simulink model "scheme2"  (R2024a)
settings: Solver=VariableStepAuto  StartTime=0.0  StopTime=10.0  RelTol=1e-8
values from neighbouring files (symbols this model uses):
  A = [8, 1, 11; 4, 0, 4; -4, -3, -7]    [main.m]
  B = [-1; -3; 3]    [main.m]
  Cz = [-2, -3, -1]    [main.m]
  Dz = [8, -8, 12, -3]    [main.m]
  Gamma = [-40, 16, 9, 7; -64, 25, 14, 12; -26, 11, 7, 3; -48, 18, 14, 8]    [main.m]
  K1 = [0, 0, 0]    [main.m]
  K2 = FindFeedforwardController(A, B, Gamma, Cz, Dz, zeros(3, 4), K1)    [main.m]
  wgen = 1    [main.m]
  x0 = [1; 1; 1]    [main.m]
settings Model: Creator=alexivanov  LastModifiedBy=alexivanov

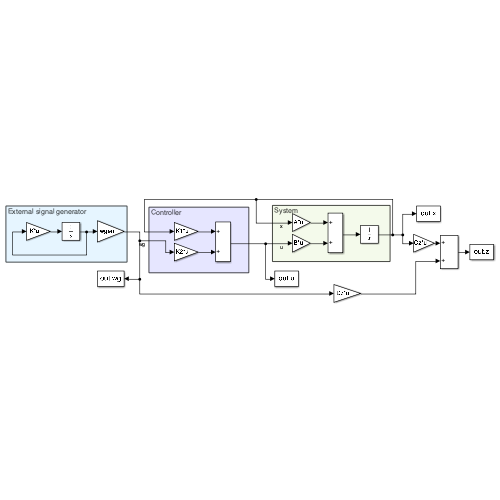
[thumbnail: Simulink's stored preview of the top-level diagram]
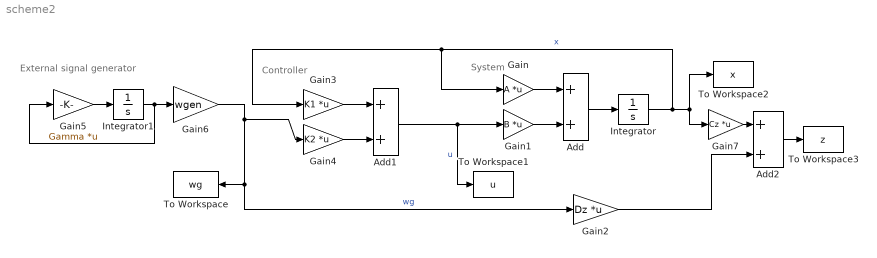
== system scheme2 ==
  note: Controller
  note: External signal generator
  note: System
  Add : Sum
  Add1 : Sum
  Add2 : Sum
  Gain : Gain  Gain=A  Multiplication=Matrix(K*u)
  Gain1 : Gain  Gain=B  Multiplication=Matrix(K*u)
  Gain2 : Gain  Gain=Dz  Multiplication=Matrix(K*u)
  Gain3 : Gain  Gain=K1  Multiplication=Matrix(K*u)
  Gain4 : Gain  Gain=K2  Multiplication=Matrix(K*u)
  Gain5 : Gain  Gain=Gamma  Multiplication=Matrix(K*u)
  Gain6 : Gain  Gain=wgen
  Gain7 : Gain  Gain=Cz  Multiplication=Matrix(K*u)
  Integrator : Integrator  InitialCondition=x0
  Integrator1 : Integrator  InitialCondition=[1; 1; 1; 1]
  To Workspace : ToWorkspace  VariableName=wg  SampleTime=-1
  To Workspace1 : ToWorkspace  VariableName=u  SampleTime=-1
  To Workspace2 : ToWorkspace  VariableName=x  SampleTime=-1
  To Workspace3 : ToWorkspace  VariableName=z  SampleTime=-1
  wires:
  Add/1 -> Integrator/1
  Gain/1 -> Add/1
  Integrator/1 -> Gain7/1, To Workspace2/1, Gain3/1, Gain/1  "x"
  Integrator1/1 -> Gain5/1, Gain6/1
  Gain6/1 -> Gain4/1, Gain2/1, To Workspace/1  "wg"
  Gain3/1 -> Add1/1
  Gain4/1 -> Add1/2
  Gain5/1 -> Integrator1/1
  Add1/1 -> To Workspace1/1, Gain1/1  "u"
  Gain1/1 -> Add/2
  Gain7/1 -> Add2/1
  Add2/1 -> To Workspace3/1
  Gain2/1 -> Add2/2
